simulink model "receptor"  (R2023b)
settings: Solver=VariableStepAuto  StartTime=0.0  StopTime=0.1  RelTol=1e-3
values from neighbouring files (symbols this model uses):
  fc1_mux = f_portadoras(1)    [simulink_parametros.m]
  fc1_receptor = frecuencia_intermedia + fc3_mux    (= 140000)    [simulink_parametros.m]
  fc2_mux = f_portadoras(2)    [simulink_parametros.m]
  fc2_receptor = frecuencia_intermedia + fc2_mux    (= 130000)    [simulink_parametros.m]
  fc3_mux = f_portadoras(3)    [simulink_parametros.m]
  fc3_receptor = frecuencia_intermedia + fc1_mux    (= 120000)    [simulink_parametros.m]
  fm1_mux = 1e3    (= 1000)    [simulink_parametros.m]
  fm2_mux = 2e3    (= 2000)    [simulink_parametros.m]
  fm3_mux = 3e3    (= 3000)    [simulink_parametros.m]
  frecuencia_intermedia = 110e3    (= 110000)    [simulink_parametros.m]
  fs_mux = 10 * frecuencia_intermedia    (= 1100000)    [simulink_parametros.m]
  ts_mux = 1/fs_mux    (= 3.33333333333e-06)    [simulink_parametros.m]
undefined symbols (not defined in the file or in its folder): am2
libraries: commanapbnd3 x5, commchan3 x1
settings Model: Creator=RomaW11  LastModifiedBy=RomaW11

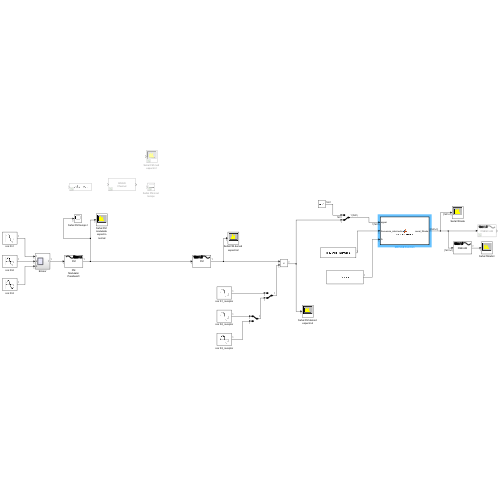
[thumbnail: Simulink's stored preview of the top-level diagram]
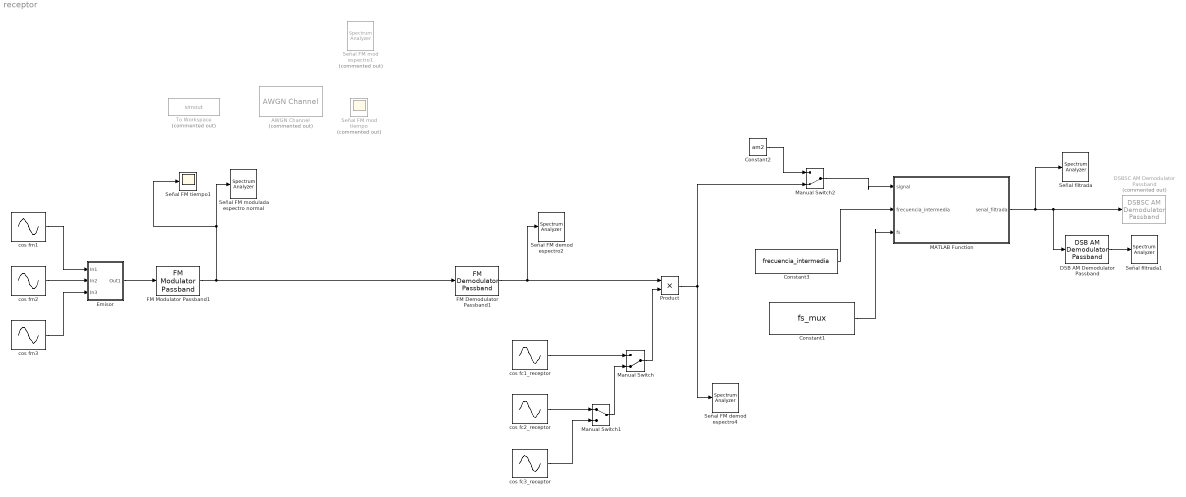
== system receptor ==
  AWGN Channel : commchan3/AWGN Channel  Commented=on  LegacyMode=off  NoiseMethod="Signal to noise ratio  (SNR)"  noiseMode="Signal to noise ratio  (SNR)"  EbNo=10  EsNo=10  SNR=10  BitsPerSymbol=1  SignalPower=1  SamplesPerSymbol=1  SymbolPeriod=1  VarianceSource=Parameter  Variance=1  RandomStream=Global stream  Seed=67  SimulateUsing=Code generation
  Constant1 : Constant  Value=fs_mux  SampleTime=ts_mux
  Constant2 : Constant  Value=am2  SampleTime=ts_mux
  Constant3 : Constant  Value=frecuencia_intermedia  SampleTime=ts_mux
  DSB AM Demodulator Passband : commanapbnd3/DSB AM Demodulator Passband  Fc=300  Ph=0  method=Butterworth  n=4  cf=300  Rp=0.1  Rs=50  Offset=1
  DSBSC AM Demodulator Passband : commanapbnd3/DSBSC AM Demodulator Passband  Commented=on  Fc=10e3  Ph=0  method=Butterworth  n=4  cf=1e3  Rp=0.1  Rs=50
  Emisor : Subsystem
  FM Demodulator Passband1 : commanapbnd3/FM Demodulator Passband  Fc=fc_mod_fm  Ph=0  Kc=50  Ho=100
  FM Modulator Passband1 : commanapbnd3/FM Modulator Passband  Fc=fc_mod_fm  Ph=0  Kc=50
  MATLAB Function : MATLAB Function  TreatAsAtomicUnit=on
  Manual Switch : ManualSwitch  CurrentSetting=0
  Manual Switch1 : ManualSwitch
  Manual Switch2 : ManualSwitch  CurrentSetting=0
  Product : Product
  Señal FM modulada espectro normal : SpectrumAnalyzer  WindowPosition=[1.000000,1.000000,1920.000000,1057.000000,]  ScopeFrameLocation=window  SampleRate=44.1e3  StartFrequency=20  StopFrequency=20e3  YLimits=[-70.08644135,31.95491239]  ShowLegend=on
      settings: OpenAtSimulationStart=off
  Señal FM demod espectro2 : SpectrumAnalyzer  WindowPosition=[1.000000,1.000000,1920.000000,1057.000000,]  ScopeFrameLocation=window  SampleRate=44.1e3  StartFrequency=20  StopFrequency=20e3  YLimits=[-74.21752509,28.04627782]  ShowLegend=on
      settings: OpenAtSimulationStart=off
  Señal FM demod espectro4 : SpectrumAnalyzer  WindowPosition=[1.000000,1.000000,1920.000000,1057.000000,]  ScopeFrameLocation=window  SampleRate=44.1e3  StartFrequency=20  StopFrequency=20e3  YLimits=[-83.26874486,22.41218057]  ShowLegend=on
      settings: OpenAtSimulationStart=off
  Señal FM mod espectro1 : SpectrumAnalyzer  Commented=on  WindowPosition=[1.000000,1.000000,1920.000000,1057.000000,]  ScopeFrameLocation=window  SampleRate=44.1e3  StartFrequency=20  StopFrequency=20e3  YLimits=[-242.03109493,52.7559722]  ShowLegend=on
      settings: OpenAtSimulationStart=off
  Señal FM mod tiempo : Scope  Commented=on
  Señal FM tiempo1 : Scope
  Señal filtrada : SpectrumAnalyzer  WindowPosition=[1.000000,1.000000,1920.000000,1057.000000,]  ScopeFrameLocation=window  SampleRate=44.1e3  Span=5000  CenterFrequency=100000  StartFrequency=95000  StopFrequency=20e3  YLimits=[-310.10641751,-6.50367955]  ShowLegend=on
      settings: OpenAtSimulationStart=off
  Señal filtrada1 : SpectrumAnalyzer  WindowPosition=[1.000000,1.000000,1920.000000,1057.000000,]  ScopeFrameLocation=window  SampleRate=44.1e3  Span=5000  CenterFrequency=100000  StartFrequency=95000  StopFrequency=20e3  YLimits=[-310.10641751,-6.50367955]  ShowLegend=on
      settings: OpenAtSimulationStart=off
  To Workspace : ToWorkspace  Commented=on  VariableName=simout  SaveFormat=Timeseries  SampleTime=-1
  cos fc1_receptor : Sin  Frequency=2*pi*fc1_receptor  Phase=pi/2  SampleTime=ts_mux
  cos fc2_receptor : Sin  Frequency=2*pi*fc2_receptor  Phase=pi/2  SampleTime=ts_mux
  cos fc3_receptor : Sin  Frequency=2*pi*fc3_receptor  Phase=pi/2  SampleTime=ts_mux
  cos fm1 : Sin  Frequency=2*pi*fm1_mux  Phase=pi/2  SampleTime=ts_mux
  cos fm2 : Sin  Frequency=2*pi*fm2_mux  Phase=pi/2  SampleTime=ts_mux
  cos fm3 : Sin  Frequency=2*pi*fm3_mux  Phase=pi/2  SampleTime=ts_mux
  wires:
  cos fm1/1 -> Emisor/1(In1)
  cos fm2/1 -> Emisor/2(In2)
  cos fm3/1 -> Emisor/3(In3)
  Manual Switch/1 -> Product/2
  cos fc1_receptor/1 -> Manual Switch/1
  cos fc2_receptor/1 -> Manual Switch1/1
  cos fc3_receptor/1 -> Manual Switch1/2
  Manual Switch1/1 -> Manual Switch/2
  Product/1 -> Manual Switch2/2, Señal FM demod espectro4/1
  MATLAB Function/1(senal_filtrada) -> DSB AM Demodulator Passband/1, DSBSC AM Demodulator Passband/1, Señal filtrada/1
  FM Demodulator Passband1/1 -> Product/1, Señal FM demod espectro2/1
  Constant1/1 -> MATLAB Function/3(fs)
  Constant3/1 -> MATLAB Function/2(frecuencia_intermedia)
  Constant2/1 -> Manual Switch2/1
  Manual Switch2/1 -> MATLAB Function/1(signal)
  FM Modulator Passband1/1 -> FM Demodulator Passband1/1, Señal FM modulada espectro normal/1, Señal FM tiempo1/1
  Emisor/1(Out1) -> FM Modulator Passband1/1
  DSB AM Demodulator Passband/1 -> Señal filtrada1/1

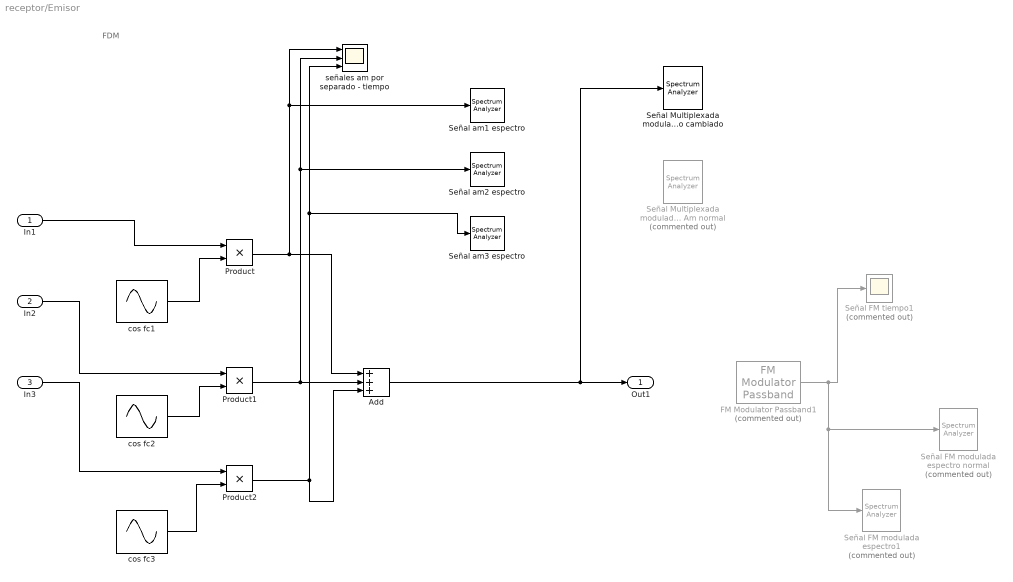
== system receptor/Emisor ==
  note: FDM
  In1 : Inport
  In2 : Inport  Port=2
  In3 : Inport  Port=3
  Add : Sum  Inputs=+++
  FM Modulator Passband1 : commanapbnd3/FM Modulator Passband  Commented=on  Fc=fc_mod_fm  Ph=0  Kc=50
  Product : Product
  Product1 : Product
  Product2 : Product
  Señal FM modulada espectro normal : SpectrumAnalyzer  Commented=on  WindowPosition=[1.000000,1.000000,1920.000000,1057.000000,]  ScopeFrameLocation=window  SampleRate=44.1e3  StartFrequency=20  StopFrequency=20e3  YLimits=[-70.25355511,31.96587949]  ShowLegend=on
      settings: OpenAtSimulationStart=off
  Señal FM modulada espectro1 : SpectrumAnalyzer  Commented=on  WindowPosition=[1.000000,1.000000,1920.000000,1057.000000,]  ScopeFrameLocation=window  SampleRate=44.1e3  StartFrequency=20  StopFrequency=20e3  YLimits=[-70.25355511,31.96587949]  ShowLegend=on  SelectedToolstripTab=spectrumAnalyzerToolstrip.measurementsTab
      settings: OpenAtSimulationStart=off
  Señal FM tiempo1 : Scope  Commented=on
  Señal Multiplexada modulada Am normal : SpectrumAnalyzer  Commented=on  WindowPosition=[1.000000,1.000000,1920.000000,1057.000000,]  ScopeFrameLocation=window  SampleRate=44.1e3  FrequencySpan=Start and stop frequencies  StartFrequency=-100000  StopFrequency=100000  Title=Señal modulada Am Multiplexada  YLimits=[-47.12602012,24.33805113]  ShowLegend=on  SelectedToolstripTab=spectrumAnalyzerToolstrip.estimationTab
      settings: OpenAtSimulationStart=off
  Señal Multiplexada modulada Am rango del espectro cambiado : SpectrumAnalyzer  WindowPosition=[1.000000,1.000000,1920.000000,1057.000000,]  ScopeFrameLocation=window  SampleRate=44.1e3  FrequencySpan=Start and stop frequencies  StartFrequency=-100000  StopFrequency=100000  Title=Señal modulada Am Multiplexada  YLimits=[-35.60353052,49.21514085]  ShowLegend=on  SelectedToolstripTab=spectrumAnalyzerToolstrip.estimationTab
      settings: OpenAtSimulationStart=off
  Señal am1 espectro : SpectrumAnalyzer  WindowPosition=[7.000000,-1079.000000,1920.000000,1057.000000,]  ScopeFrameLocation=window  SampleRate=44.1e3  StartFrequency=20  StopFrequency=20e3  YLimits=[-217.97153023,70.59577818]  ShowLegend=on
      settings: OpenAtSimulationStart=off
  Señal am2 espectro : SpectrumAnalyzer  WindowPosition=[7.000000,-1079.000000,1920.000000,1057.000000,]  ScopeFrameLocation=window  SampleRate=44.1e3  StartFrequency=20  StopFrequency=20e3  YLimits=[-241.38361848,46.7073144]  ShowLegend=on
      settings: OpenAtSimulationStart=off
  Señal am3 espectro : SpectrumAnalyzer  WindowPosition=[7.000000,-1079.000000,1920.000000,1057.000000,]  ScopeFrameLocation=window  SampleRate=44.1e3  StartFrequency=20  StopFrequency=20e3  YLimits=[-241.50271277,46.78785835]  ShowLegend=on  ExpandToolstrip=on
      settings: OpenAtSimulationStart=off
  cos fc1 : Sin  Frequency=2*pi*fc1_mux  Phase=pi/2  SampleTime=ts_mux
  cos fc2 : Sin  Frequency=2*pi*fc2_mux  Phase=pi/2  SampleTime=ts_mux
  cos fc3 : Sin  Frequency=2*pi*fc3_mux  Phase=pi/2  SampleTime=ts_mux
  señales am por separado - tiempo : Scope  NumInputPorts=3
  Out1 : Outport
  wires:
  Add/1 -> Out1/1, Señal Multiplexada modulada Am rango del espectro cambiado/1
  FM Modulator Passband1/1 -> Señal FM modulada espectro1/1, Señal FM modulada espectro normal/1, Señal FM tiempo1/1
  In3/1 -> Product2/1
  cos fc1/1 -> Product/2
  Product1/1 -> Señal am2 espectro/1, señales am por separado - tiempo/2, Add/2
  Product/1 -> Señal am1 espectro/1, señales am por separado - tiempo/1, Add/1
  In2/1 -> Product1/1
  In1/1 -> Product/1
  cos fc2/1 -> Product1/2
  Product2/1 -> Add/3, señales am por separado - tiempo/3, Señal am3 espectro/1
  cos fc3/1 -> Product2/2

== matlab function receptor/MATLAB Function ==
  data: senal_filtrada output; signal input; frecuencia_intermedia input; fs input
function senal_filtrada = filtroPasoBanda(signal, frecuencia_intermedia, fs)
    % Filtro Paso Banda
    % Crea un filtro paso banda Butterworth para aislar un tono en la FI.
    %
    % Entradas:
    %   f_central   - Frecuencia central del tono a filtrar (en Hz)
    %   ancho_banda - Ancho de banda del filtro (en Hz)
    %   fs          - Frecuencia de muestreo de la señal (en Hz)
    %
    % Salidas:
    %   b, a - Coeficientes del filtro paso banda

    % Calcular las frecuencias de corte del filtro paso banda
    ancho_banda = 10e3;
    f1 = (frecuencia_intermedia) - (ancho_banda / 2);
    f2 = (frecuencia_intermedia) + (ancho_banda / 2);

    % Convertir las frecuencias de corte a frecuencias normalizadas (0 a 1)
    Wn = [f1 f2] / (fs / 2);

    % Orden del filtro (ajusta si es necesario)
    orden = 4;

    % Diseño del filtro Butterworth paso banda
    [b, a] = butter(orden, Wn, 'bandpass');
    senal_filtrada = filter(b, a, signal);
    senal_filtrada = senal_filtrada{1};
end
